simulink model "LQR"  (R2025b)
settings: Solver=FixedStepAuto  StartTime=0.0  StopTime=20  FixedStep=0.01  RelTol=1e-3
settings Model: Creator=flyin  LastModifiedBy=flyin
settings SolverCC: EnableFixedStepZeroCrossing=on  MaxZcPerStep=10.0

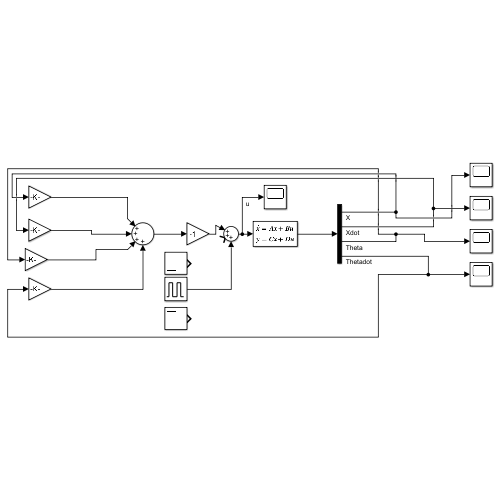
[thumbnail: Simulink's stored preview of the top-level diagram]
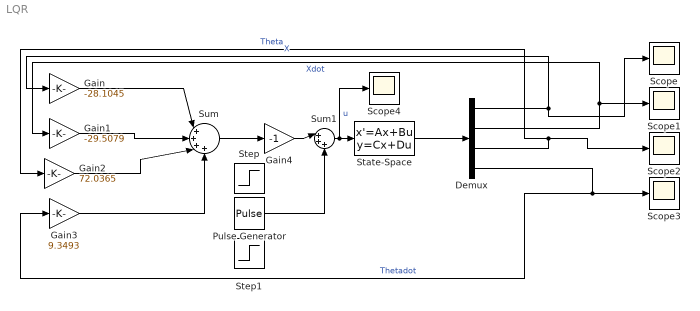
== system LQR ==
  Demux : Demux
  Gain : Gain  Gain=-28.1045
  Gain1 : Gain  Gain=-29.5079
  Gain2 : Gain  Gain=72.0365
  Gain3 : Gain  Gain=9.3493
  Gain4 : Gain  Gain=-1
  Pulse Generator : DiscretePulseGenerator  PulseType=Time based  Amplitude=-6  Period=100  PulseWidth=0.05
  Scope{,1..4} (5 alike) : Scope
      Scope settings: ActiveDisplayYMinimum=-0.33896225819838038  ActiveDisplayYMaximum=0.054310335687515268  YLabel=meter  DataLoggingVariableName=lqrX  DataLoggingSaveFormat=Array
      Scope1 settings: ActiveDisplayYMinimum=-0.532777097767577  ActiveDisplayYMaximum=0.15004831099697646
      Scope2 settings: ActiveDisplayYMinimum=-0.12728693159279558  ActiveDisplayYMaximum=0.12728693100088423  YLabel=theta  DataLoggingVariableName=lqrTheta  DataLoggingSaveFormat=Array
      Scope3 settings: DataLoggingVariableName=ScopeData3
      Scope4 settings: ActiveDisplayYMinimum=-10.000000016672745  ActiveDisplayYMaximum=10.000000001852527  YLabel=U  DataLoggingVariableName=lqrU  DataLoggingSaveFormat=Array
  State-Space : StateSpace  A=|  B=|  C=[1.0 0.0 0.0 0.0; 0.0 1.0 0.0 0.0; 0.0 0.0 1.0 0.0; 0.0 0.0 0.0 1.0]  D=[0.0; 0.0; 0.0; 0.0]  InitialCondition=[0.013388091; 0.0; 0; 0]
      A=|
      | [    0    1.0000         0         0
      |  ;        0  -10.0000    1.6498   -0.0137
      |   ;  0   0  0  1.0000 ;0  -57.1429   65.5415   -0.5448]
      B=|
      | [0
      |  ;   2.0000
      |   ;       0
      |  ;  -11.4286]
  Step : Step  Time=0  After=8  SampleTime=0
  Step1 : Step  Time=10  After=-8  SampleTime=0
  Sum : Sum  Inputs=|++++
  Sum1 : Sum  Inputs=|+++
  wires:
  State-Space/1 -> Demux/1
  Demux/1 -> Gain/1, Scope/1  "X"
  Demux/2 -> Gain1/1, Scope1/1  "Xdot"
  Demux/3 -> Gain2/1, Scope2/1  "Theta"
  Demux/4 -> Gain3/1, Scope3/1  "Thetadot"
  Sum/1 -> Gain4/1
  Gain3/1 -> Sum/4
  Gain2/1 -> Sum/3
  Gain1/1 -> Sum/2
  Gain/1 -> Sum/1
  Gain4/1 -> Sum1/1
  Sum1/1 -> Scope4/1, State-Space/1  "u"
  Pulse Generator/1 -> Sum1/3
